simulink model "NavFilterTestHarness24"  (R2016b)
settings: Solver=FixedStepDiscrete  StartTime=startTime  StopTime=endTime  FixedStep=0.001  RelTol=1e-3  EnableMultiTasking=on
undefined symbols (not defined in the file): accel, ADSframe, ADStime, alignTime, angRate, ATTframe, CourseDeg, EAS2TAS, GndSpd, GPSframe, GPStime, Hgt, IMUframe, IMUtime, LatDeg, LngDeg, MagBiasX, MagBiasY, MagBiasZ, MAGframe, MAGtime, MagX, MagY, MagZ, msecHgtDelay, msecMagDelay, msecPosDelay, msecTasDelay, msecVelDelay, Pitch, Roll, Veas, VelD, Yaw
libraries: simulink x9, simulink_need_slupdate x2
(part 1 of 5)
settings Model: SimulationMode=rapid-accelerator  ExtModeTrigDuration=100  Creator=user  LastModifiedBy=lizarraga
settings DataIOCC: LimitDataPoints=on  SaveFinalState=on  SaveFormat=Array  SignalLoggingSaveFormat=ModelDataLogs  SaveOutput=off  SaveState=on  StateSaveName=tmp_raccel_xout
settings OptimizationCC: ExpressionDepthLimit=2147483647  EfficientMapNaN2IntZero=off  LifeSpan=inf
settings DebuggingCC: CheckSSInitialOutputMsg=off  UnderspecifiedInitializationDetection=Classic  MergeDetectMultiDrivingBlocksExec=none  SolverPrmCheckMsg=warning  ParameterPrecisionLossMsg=none  StateNameClashWarn=warning  SFUnexpectedBacktrackingDiag=warning  SFNoUnconditionalDefaultTransitionDiag=warning  SFExecutionAtInitializationDiag=none
settings HardwareCC: ProdBitPerPointer=32  ProdBitPerSizeT=32  ProdBitPerPtrDiffT=32  ProdLargestAtomicFloat=None  ProdIntDivRoundTo=Undefined  ProdEndianess=Unspecified  ProdWordSize=32  ProdHWDeviceType=32-bit Generic  TargetBitPerLong=64  TargetBitPerPointer=64  TargetBitPerSizeT=64  TargetBitPerPtrDiffT=64  TargetLongLongMode=on  TargetIntDivRoundTo=Zero  TargetEndianess=LittleEndian  TargetWordSize=64  TargetHWDeviceType=MATLAB Host  ProdEqTarget=off
settings ModelReferenceCC: PropagateSignalLabelsOutOfModel=off
settings SFSimCC: SimParseCustomCode=off
settings RTWCC: SystemTargetFile=raccel.tlc  TemplateMakefile=raccel_default_tmf  RTWVerbose=off  RTWUseSimCustomCode=on
settings CodeAppCC: GenerateComments=off  MaxIdLength=128  SimulinkBlockComments=off
settings RaccelTargetCC: ERTMultiwordTypeDef=System defined  ERTMultiwordLength=256  ParMdlRefBuildCompliant=off  GeneratePreprocessorConditionals=Disable all  ERTFirstTimeCompliant=off  MultiInstanceERTCode=off  ENABLE_SLEXEC_SSBRIDGE=0  RTWCAPISignals=off  RTWCAPIParams=off
settings ConfigComp: CovMetricSettings=dw  CovHtmlReporting=on  CovSaveCumulativeToWorkspaceVar=on  CovSaveSingleToWorkspaceVar=on  CovExternalEMLEnable=off

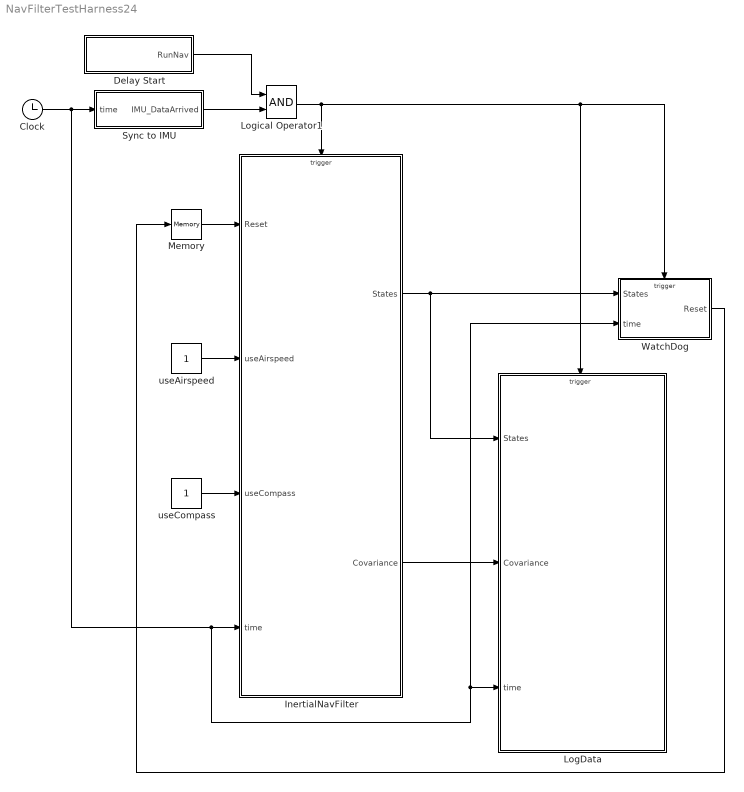
== system NavFilterTestHarness24 ==
  Clock : Clock
  Delay Start : Subsystem  TreatAsAtomicUnit=on  mask{navStartTime=alignTime}
      mask prompts: navStartTime "Nav Start Time"
  InertialNavFilter : Subsystem
  LogData : Subsystem
  Logical Operator1 : Logic  AllPortsSameDT=off  OutDataTypeStr=boolean
  Memory : Memory  InheritSampleTime=on
  Sync to IMU : Subsystem  TreatAsAtomicUnit=on
  WatchDog : Subsystem  TreatAsAtomicUnit=on
  useAirspeed : Constant  OutDataTypeStr=boolean
  useCompass : Constant  OutDataTypeStr=boolean
  wires:
  InertialNavFilter/1(States) -> LogData/1(States), WatchDog/1(States)
  Logical Operator1/1 -> LogData/Trigger, WatchDog/Trigger, InertialNavFilter/Trigger
  InertialNavFilter/2(Covariance) -> LogData/2(Covariance)
  WatchDog/1(Reset) -> Memory/1
  useAirspeed/1 -> InertialNavFilter/2(useAirspeed)
  useCompass/1 -> InertialNavFilter/3(useCompass)
  Clock/1 -> InertialNavFilter/4(time), LogData/3(time), WatchDog/2(time), Sync to IMU/1(time)
  Delay Start/1(RunNav) -> Logical Operator1/1
  Sync to IMU/1(IMU_DataArrived) -> Logical Operator1/2
  Memory/1 -> InertialNavFilter/1(Reset)

== system NavFilterTestHarness24/Delay Start ==
  Clock : Clock
  Compare To Constant2 : simulink/Logic and Bit Operations/Compare To Constant  relop=>  const=navStartTime  OutDataTypeStr=boolean
  RunNav : Outport
  wires:
  Clock/1 -> Compare To Constant2/1
  Compare To Constant2/1 -> RunNav/1

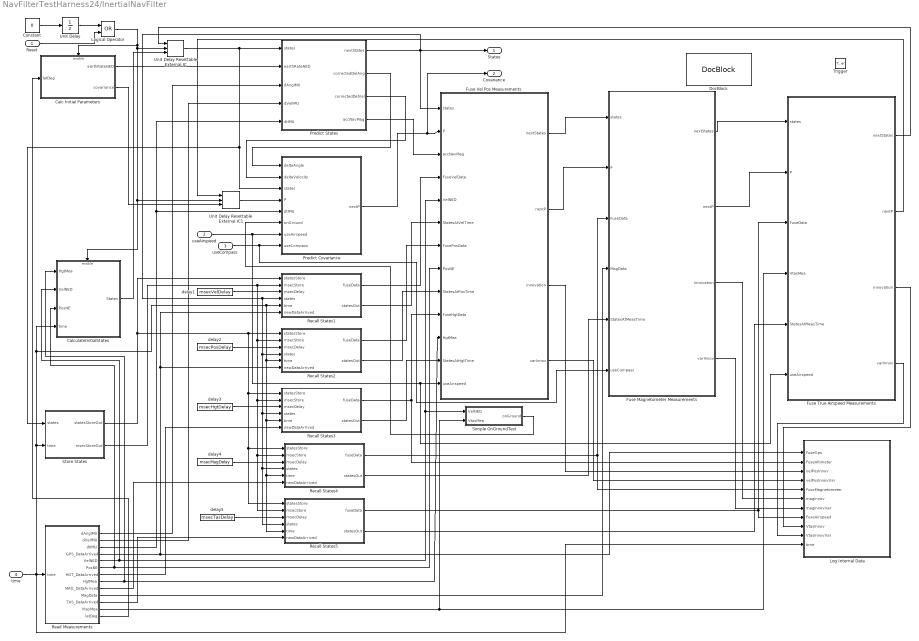
== system NavFilterTestHarness24/InertialNavFilter ==
  Reset : Inport  OutDataTypeStr=boolean  PortDimensions=1
  useAirspeed : Inport  Port=2  OutDataTypeStr=boolean  PortDimensions=1
  useCompass : Inport  Port=3  OutDataTypeStr=boolean  PortDimensions=1
  time : Inport  Port=4  OutDataTypeStr=double  PortDimensions=1
  Trigger : TriggerPort  VariantControl=Variant  PortDimensions=1
  Calc Initial Parameters : Subsystem
  CalculateInitialStates : Subsystem  TreatAsAtomicUnit=on
  Constant : Constant  Value=0  OutDataTypeStr=boolean
  DocBlock : simulink/Model-Wide Utilities/DocBlock  DocumentType=Text
      content=|
      | 24 State Extended Kalman Filter
      |
      | States :
      | 1 ... 4   : Quaternion parameters defining the rotation from local NED tangent frame to XYZ body axes
      | 5 ... 7   : North, East, Down velocity relative to and earth fixed reference point (m)
      | 8 ... 10  : North, East, Down position relative to and earth fixed reference point (m)
      | 11 ... 13 : IMU delta angle bias errors (rad)
      | 14 ... 16 : IMU delta velocity bias errors (m/s)
      | 17,18     : North, East wind velocity (m/s)
      | 19 ... 21 : North, East, Down earth magnetic field (same units as magnetometer output)
      | 22 ... 24 : X, Y, Z Body fixed magnetic field bias - opposite sign to APM offsets (same units as magnetometer output)
      |
      | Time Varying Parameters :
      | IMU delta angles (rad)
      | IMU delta velocity (rad)
      |
      | Observations :
      | North, East, Down velocity (m/s)
      | North, East position (m)
      | Height (m)
      | True Airspeed (m/s) - optional
      | X, Y, Z body fixed magnetic flux measurements (same units as magnetometer output) - optional
      |
      | Note : without compass/magnetometer measurements, the heading alignment cannot be maintained on the ground, so the filter will need to be re-started when flight commences.
  Fuse Magnetometer Measurements : MATLAB Function  TreatAsAtomicUnit=on
  Fuse True Airspeed Measurements : MATLAB Function  TreatAsAtomicUnit=on
  Fuse Vel Pos Measurements : MATLAB Function  TreatAsAtomicUnit=on
  Log Internal Data : Subsystem
  Logical Operator : Logic  Operator=OR  AllPortsSameDT=off  OutDataTypeStr=boolean
  Predict Covariance : MATLAB Function  TreatAsAtomicUnit=on
  Predict States : MATLAB Function  TreatAsAtomicUnit=on
  Read Measurements : Subsystem  TreatAsAtomicUnit=on
  Recall States1 : MATLAB Function  TreatAsAtomicUnit=on
  Recall States2 : MATLAB Function  TreatAsAtomicUnit=on
  Recall States3 : MATLAB Function  TreatAsAtomicUnit=on
  Recall States4 : MATLAB Function  TreatAsAtomicUnit=on
  Recall States5 : MATLAB Function  TreatAsAtomicUnit=on
  Simple OnGroundTest : Subsystem  TreatAsAtomicUnit=on
  Store States : MATLAB Function  TreatAsAtomicUnit=on
  Unit Delay : UnitDelay  InitialCondition=1  SampleTime=-1
  Unit Delay Resettable External IC : simulink_need_slupdate/Unit Delay Resettable External IC  tsamp=-1
  Unit Delay Resettable External IC1 : simulink_need_slupdate/Unit Delay Resettable External IC  tsamp=-1
  delay1 : Constant  Value=msecVelDelay  OutDataTypeStr=int32  SampleTime=-1
  delay2 : Constant  Value=msecPosDelay  OutDataTypeStr=int32  SampleTime=-1
  delay3 : Constant  Value=msecHgtDelay  OutDataTypeStr=int32  SampleTime=-1
  delay4 : Constant  Value=msecMagDelay  OutDataTypeStr=int32  SampleTime=-1
  delay5 : Constant  Value=msecTasDelay  OutDataTypeStr=int32  SampleTime=-1
  States : Outport  OutDataTypeStr=single  PortDimensions=24
  Covariance : Outport  Port=2  OutDataTypeStr=single  PortDimensions=[24,24]
  wires:
  CalculateInitialStates/1(States) -> Unit Delay Resettable External IC/3
  Unit Delay Resettable External IC/1 -> Predict States/1(states), Predict Covariance/3(states), Store States/1(states)
  Predict States/1(nextStates) -> States/1, Fuse Vel Pos Measurements/1(states), Recall States1/4(states), Recall States2/4(states), Recall States5/4(states), Recall States4/4(states), Recall States3/4(states)
  Unit Delay Resettable External IC1/1 -> Predict Covariance/4(P)
  Calc Initial Parameters/2(covariance) -> Unit Delay Resettable External IC1/3
  Predict States/2(correctedDelAng) -> Predict Covariance/1(deltaAngle)
  Predict States/3(correctedDelVel) -> Predict Covariance/2(deltaVelocity)
  Fuse Vel Pos Measurements/2(nextP) -> Fuse Magnetometer Measurements/2(P)
  Fuse Vel Pos Measurements/1(nextStates) -> Fuse Magnetometer Measurements/1(states)
  Fuse True Airspeed Measurements/2(nextP) -> Unit Delay Resettable External IC1/1
  Fuse True Airspeed Measurements/1(nextStates) -> Unit Delay Resettable External IC/1
  Fuse Magnetometer Measurements/1(nextStates) -> Fuse True Airspeed Measurements/1(states)
  Fuse Magnetometer Measurements/2(nextP) -> Fuse True Airspeed Measurements/2(P)
  Predict Covariance/1(nextP) -> Covariance/1, Fuse Vel Pos Measurements/2(P)
  Predict States/4(accNavMag) -> Fuse Vel Pos Measurements/3(accNavMag)
  Unit Delay/1 -> Logical Operator/1
  useCompass/1 -> Predict Covariance/8(useCompass), Fuse Magnetometer Measurements/6(useCompass)
  useAirspeed/1 -> Predict Covariance/7(useAirspeed), Fuse Vel Pos Measurements/13(useAirspeed), Fuse True Airspeed Measurements/6(useAirspeed)
  Fuse True Airspeed Measurements/3(innovation) -> Log Internal Data/9(VtasInnov)
  Fuse True Airspeed Measurements/4(varInnov) -> Log Internal Data/10(VtasInnovVar)
  Fuse Magnetometer Measurements/3(innovation) -> Log Internal Data/6(magInnov)
  Fuse Vel Pos Measurements/3(innovation) -> Log Internal Data/3(velPosInnov)
  Fuse Magnetometer Measurements/4(varInnov) -> Log Internal Data/7(magInnovVar)
  Fuse Vel Pos Measurements/4(varInnov) -> Log Internal Data/4(velPosInnovVar)
  time/1 -> Read Measurements/1(time), Log Internal Data/11(time), Store States/2(time), CalculateInitialStates/4(time), Recall States1/5(time), Recall States2/5(time), Recall States3/5(time), Recall States5/5(time), Recall States4/5(time)
  Simple OnGroundTest/1(onGround) -> Predict Covariance/6(onGround)
  Read Measurements/4(GPS_DataArrived) -> Log Internal Data/1(FuseGps), Recall States1/6(newDataArrived), Recall States2/6(newDataArrived)
  Read Measurements/5(VelNED) -> Simple OnGroundTest/1(VelNED), Fuse Vel Pos Measurements/5(VelNED), CalculateInitialStates/2(VelNED)
  Read Measurements/6(PosNE) -> CalculateInitialStates/3(PosNE), Fuse Vel Pos Measurements/8(PosNE)
  Read Measurements/8(HgtMea) -> CalculateInitialStates/1(HgtMea), Fuse Vel Pos Measurements/11(HgtMea)
  Read Measurements/10(MagData) -> Fuse Magnetometer Measurements/4(MagData)
  Read Measurements/12(VtasMea) -> Fuse True Airspeed Measurements/4(VtasMea), Simple OnGroundTest/2(VtasMea)
  Read Measurements/13(latDeg) -> Calc Initial Parameters/1(latDeg)
  Calc Initial Parameters/1(earthRateNED) -> Predict States/2(earthRateNED)
  Read Measurements/3(dtIMU) -> Predict Covariance/5(dtIMU), Predict States/5(dtIMU)
  Constant/1 -> Unit Delay/1
  Reset/1 -> Logical Operator/2
  Read Measurements/1(dAngIMU) -> Predict States/3(dAngIMU)
  Read Measurements/2(dVelIMU) -> Predict States/4(dVelIMU)
  Logical Operator/1 -> Unit Delay Resettable External IC/2, Unit Delay Resettable External IC1/2, CalculateInitialStates/Enable, Calc Initial Parameters/Enable
  Recall States1/2(statesOut) -> Fuse Vel Pos Measurements/6(StatesAtVelTime)
  Recall States1/1(fuseData) -> Fuse Vel Pos Measurements/4(FuseVelData)
  delay1/1 -> Recall States1/3(msecDelay)
  Store States/1(statesStoreOut) -> Recall States1/1(statesStore), Recall States2/1(statesStore), Recall States3/1(statesStore), Recall States4/1(statesStore), Recall States5/1(statesStore)
  Store States/2(msecStoreOut) -> Recall States1/2(msecStore), Recall States3/2(msecStore), Recall States4/2(msecStore), Recall States5/2(msecStore), Recall States2/2(msecStore)
  delay3/1 -> Recall States3/3(msecDelay)
  delay4/1 -> Recall States4/3(msecDelay)
  delay5/1 -> Recall States5/3(msecDelay)
  delay2/1 -> Recall States2/3(msecDelay)
  Read Measurements/7(HGT_DataArrived) -> Recall States3/6(newDataArrived)
  Read Measurements/9(MAG_DataArrived) -> Recall States4/6(newDataArrived)
  Read Measurements/11(TAS_DataArrived) -> Recall States5/6(newDataArrived)
  Recall States2/1(fuseData) -> Fuse Vel Pos Measurements/7(FusePosData)
  Recall States2/2(statesOut) -> Fuse Vel Pos Measurements/9(StatesAtPosTime)
  Recall States3/1(fuseData) -> Fuse Vel Pos Measurements/10(FuseHgtData), Log Internal Data/2(FuseAltimeter)
  Recall States3/2(statesOut) -> Fuse Vel Pos Measurements/12(StatesAtHgtTime)
  Recall States4/1(fuseData) -> Fuse Magnetometer Measurements/3(FuseData), Log Internal Data/5(FuseMagnetometer)
  Recall States4/2(statesOut) -> Fuse Magnetometer Measurements/5(StatesAtMeasTime)
  Recall States5/1(fuseData) -> Fuse True Airspeed Measurements/3(FuseData), Log Internal Data/8(FuseAirspeed)
  Recall States5/2(statesOut) -> Fuse True Airspeed Measurements/5(StatesAtMeasTime)

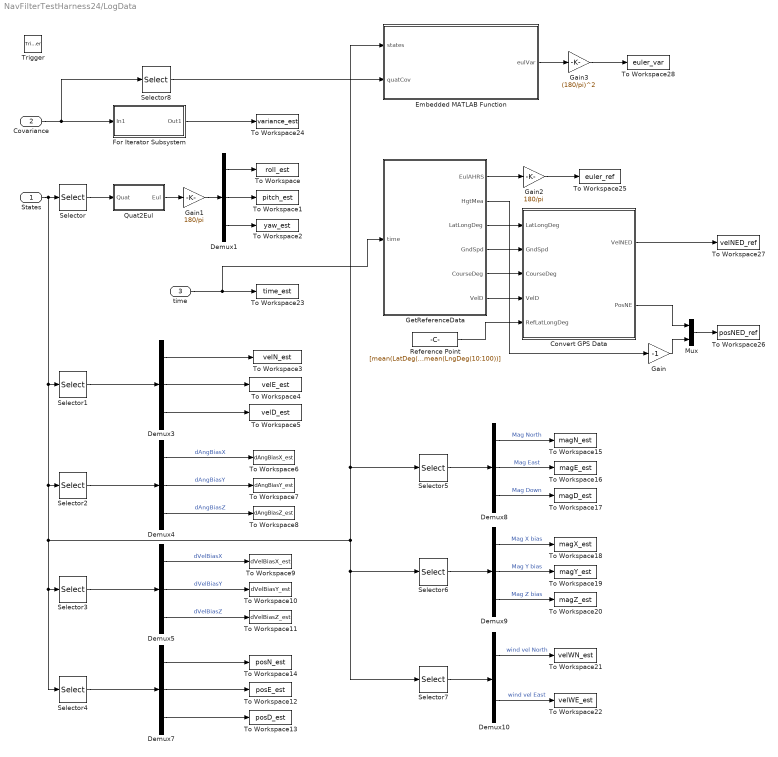
== system NavFilterTestHarness24/LogData ==
  States : Inport
  Covariance : Inport  Port=2  PortDimensions=[24,24]
  time : Inport  Port=3  OutDataTypeStr=double  PortDimensions=1
  Trigger : TriggerPort  VariantControl=Variant  PortDimensions=1
  Convert GPS Data : MATLAB Function  TreatAsAtomicUnit=on
  Demux{1,3..5,7..9} (7 alike) : Demux  Outputs=3
  Demux10 : Demux  Outputs=2
  Embedded MATLAB Function : MATLAB Function  TreatAsAtomicUnit=on
  For Iterator Subsystem : Subsystem  TreatAsAtomicUnit=on
  Gain : Gain  Gain=-1
  Gain1 : Gain  Gain=180/pi
  Gain2 : Gain  Gain=180/pi
  Gain3 : Gain  Gain=(180/pi)^2
  GetReferenceData : Subsystem  TreatAsAtomicUnit=on
  Mux : Mux  Inputs=2
  Quat2Eul : Subsystem
  Reference Point : Constant  Value=[mean(LatDeg(10:100)),mean(LngDeg(10:100))]  OutDataTypeStr=single
  Selector : Selector  InputPortWidth=24  IndexOptions=Index vector (dialog)  Indices=[1:4]  OutputSizes=1
  Selector1 : Selector  InputPortWidth=24  IndexOptions=Index vector (dialog)  Indices=[5:7]  OutputSizes=1
  Selector2 : Selector  InputPortWidth=24  IndexOptions=Index vector (dialog)  Indices=[11:13]  OutputSizes=1
  Selector3 : Selector  InputPortWidth=24  IndexOptions=Index vector (dialog)  Indices=[14:16]  OutputSizes=1
  Selector4 : Selector  InputPortWidth=24  IndexOptions=Index vector (dialog)  Indices=[8:10]  OutputSizes=1
  Selector5 : Selector  InputPortWidth=24  IndexOptions=Index vector (dialog)  Indices=[19:21]  OutputSizes=1
  Selector6 : Selector  InputPortWidth=24  IndexOptions=Index vector (dialog)  Indices=[22:24]  OutputSizes=1
  Selector7 : Selector  InputPortWidth=24  IndexOptions=Index vector (dialog)  Indices=[17:18]  OutputSizes=1
  Selector8 : Selector  NumberOfDimensions=2  InputPortWidth=3  IndexOptions=Index vector (dialog),Index vector (dialog)  Indices=[1:4],[1:4]  OutputSizes=1,1
  To Workspace : ToWorkspace  VariableName=roll_est  SampleTime=-1
  To Workspace1 : ToWorkspace  VariableName=pitch_est  SampleTime=-1
  To Workspace10 : ToWorkspace  VariableName=dVelBiasY_est  SampleTime=-1
  To Workspace11 : ToWorkspace  VariableName=dVelBiasZ_est  SampleTime=-1
  To Workspace12 : ToWorkspace  VariableName=posE_est  SampleTime=-1
  To Workspace13 : ToWorkspace  VariableName=posD_est  SampleTime=-1
  To Workspace14 : ToWorkspace  VariableName=posN_est  SampleTime=-1
  To Workspace15 : ToWorkspace  VariableName=magN_est  SampleTime=-1
  To Workspace16 : ToWorkspace  VariableName=magE_est  SampleTime=-1
  To Workspace17 : ToWorkspace  VariableName=magD_est  SampleTime=-1
  To Workspace18 : ToWorkspace  VariableName=magX_est  SampleTime=-1
  To Workspace19 : ToWorkspace  VariableName=magY_est  SampleTime=-1
  To Workspace2 : ToWorkspace  VariableName=yaw_est  SampleTime=-1
  To Workspace20 : ToWorkspace  VariableName=magZ_est  SampleTime=-1
  To Workspace21 : ToWorkspace  VariableName=velWN_est  SampleTime=-1
  To Workspace22 : ToWorkspace  VariableName=velWE_est  SampleTime=-1
  To Workspace23 : ToWorkspace  VariableName=time_est  SampleTime=-1
  To Workspace24 : ToWorkspace  VariableName=variance_est  SampleTime=-1
  To Workspace25 : ToWorkspace  VariableName=euler_ref  SampleTime=-1
  To Workspace26 : ToWorkspace  VariableName=posNED_ref  SampleTime=-1
  To Workspace27 : ToWorkspace  VariableName=velNED_ref  SampleTime=-1
  To Workspace28 : ToWorkspace  VariableName=euler_var  SampleTime=-1
  To Workspace3 : ToWorkspace  VariableName=velN_est  SampleTime=-1
  To Workspace4 : ToWorkspace  VariableName=velE_est  SampleTime=-1
  To Workspace5 : ToWorkspace  VariableName=velD_est  SampleTime=-1
  To Workspace6 : ToWorkspace  VariableName=dAngBiasX_est  SampleTime=-1
  To Workspace7 : ToWorkspace  VariableName=dAngBiasY_est  SampleTime=-1
  To Workspace8 : ToWorkspace  VariableName=dAngBiasZ_est  SampleTime=-1
  To Workspace9 : ToWorkspace  VariableName=dVelBiasX_est  SampleTime=-1
  wires:
  Quat2Eul/1(Eul) -> Gain1/1
  Selector/1 -> Quat2Eul/1(Quat)
  States/1 -> Selector2/1, Selector4/1, Selector3/1, Embedded MATLAB Function/1(states), Selector5/1, Selector6/1, Selector7/1, Selector1/1, Selector/1
  Gain1/1 -> Demux1/1
  Selector2/1 -> Demux4/1
  Selector3/1 -> Demux5/1
  Demux4/1 -> To Workspace6/1  "dAngBiasX"
  Selector4/1 -> Demux7/1
  Selector5/1 -> Demux8/1
  Selector6/1 -> Demux9/1
  Selector7/1 -> Demux10/1
  Demux4/3 -> To Workspace8/1  "dAngBiasZ"
  Demux4/2 -> To Workspace7/1  "dAngBiasY"
  Demux5/1 -> To Workspace9/1  "dVelBiasX"
  Demux5/2 -> To Workspace10/1  "dVelBiasY"
  Demux5/3 -> To Workspace11/1  "dVelBiasZ"
  Demux8/1 -> To Workspace15/1  "Mag North"
  Demux8/2 -> To Workspace16/1  "Mag East"
  Demux8/3 -> To Workspace17/1  "Mag Down"
  Demux9/1 -> To Workspace18/1  "Mag X bias"
  Demux9/2 -> To Workspace19/1  "Mag Y bias"
  Demux9/3 -> To Workspace20/1  "Mag Z bias"
  Demux10/1 -> To Workspace21/1  "wind vel North"
  Demux10/2 -> To Workspace22/1  "wind vel East"
  time/1 -> To Workspace23/1, GetReferenceData/1(time)
  Demux7/1 -> To Workspace14/1
  Demux7/2 -> To Workspace12/1
  Demux7/3 -> To Workspace13/1
  Demux3/1 -> To Workspace3/1
  Demux3/2 -> To Workspace4/1
  Demux3/3 -> To Workspace5/1
  Demux1/3 -> To Workspace2/1
  Demux1/2 -> To Workspace1/1
  Demux1/1 -> To Workspace/1
  Covariance/1 -> Selector8/1, For Iterator Subsystem/1(In1)
  GetReferenceData/1(EulAHRS) -> Gain2/1
  GetReferenceData/2(HgtMea) -> Gain/1
  Convert GPS Data/2(PosNE) -> Mux/1
  Mux/1 -> To Workspace26/1
  Gain/1 -> Mux/2
  Gain2/1 -> To Workspace25/1
  Embedded MATLAB Function/1(eulVar) -> Gain3/1
  For Iterator Subsystem/1(Out1) -> To Workspace24/1
  Selector8/1 -> Embedded MATLAB Function/2(quatCov)
  Gain3/1 -> To Workspace28/1
  Selector1/1 -> Demux3/1
  GetReferenceData/3(LatLongDeg) -> Convert GPS Data/1(LatLongDeg)
  GetReferenceData/4(GndSpd) -> Convert GPS Data/2(GndSpd)
  GetReferenceData/5(CourseDeg) -> Convert GPS Data/3(CourseDeg)
  GetReferenceData/6(VelD) -> Convert GPS Data/4(VelD)
  Reference Point/1 -> Convert GPS Data/5(RefLatLongDeg)
  Convert GPS Data/1(VelNED) -> To Workspace27/1

== system NavFilterTestHarness24/Sync to IMU ==
  time : Inport
  Detect Change1 : simulink/Logic and Bit Operations/Detect Change  vinit=0  InputProcessing=Inherited  OutDataTypeStr=boolean
  Lookup Frame Counter : Lookup_n-D  NumberOfTableDimensions=1  BreakpointsForDimension1=IMUtime  BeginIndexSearchUsingPreviousIndexResult=on  Table=IMUframe  InterpMethod=Flat  DiagnosticForOutOfRangeInput=Error  RndMeth=Simplest  InputSameDT=on
  IMU_DataArrived : Outport  OutDataTypeStr=boolean
  wires:
  Lookup Frame Counter/1 -> Detect Change1/1
  time/1 -> Lookup Frame Counter/1
  Detect Change1/1 -> IMU_DataArrived/1

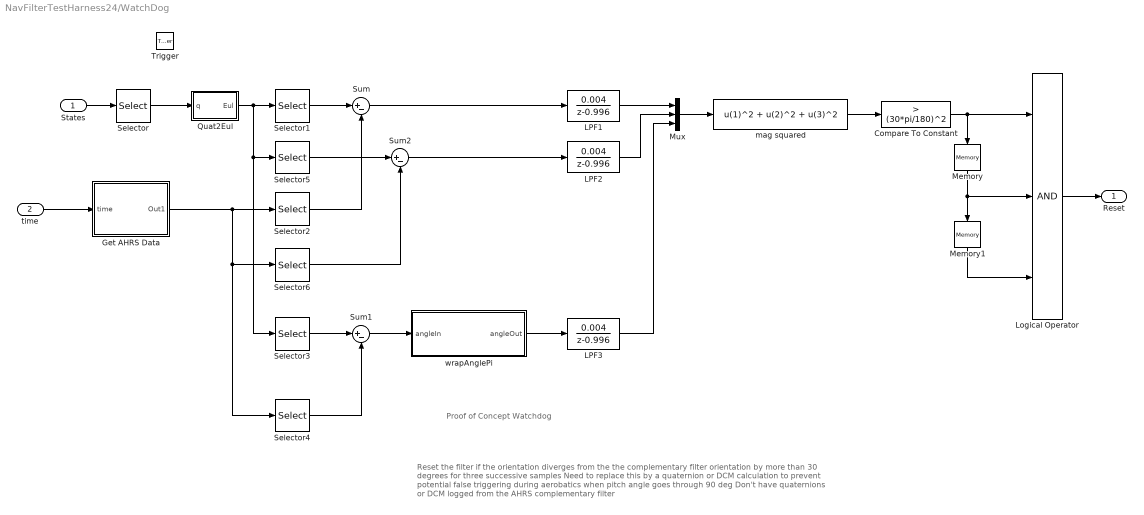
== system NavFilterTestHarness24/WatchDog ==
  note: Reset the filter if the orientation diverges from the the complementary filter orientation  by more than 30 degrees for three successive samples
      | Need to replace this by a quaternion or DCM calculation to prevent potential false triggering during aerobatics when pitch angle goes through 90 deg
      | Don't have quaternions or DCM logged from the AHRS complementary filter
  note: Proof of Concept Watchdog
  States : Inport
  time : Inport  Port=2
  Trigger : TriggerPort  VariantControl=Variant  PortDimensions=1
  Compare To Constant : simulink/Logic and Bit Operations/Compare To Constant  relop=>  const=(30*pi/180)^2  OutDataTypeStr=boolean
  Get AHRS Data : Subsystem
  LPF1 : DiscreteTransferFcn  Numerator=0.004  Denominator=[1 -0.996]
  LPF2 : DiscreteTransferFcn  Numerator=0.004  Denominator=[1 -0.996]
  LPF3 : DiscreteTransferFcn  Numerator=0.004  Denominator=[1 -0.996]
  Logical Operator : Logic  Inputs=3  AllPortsSameDT=off  OutDataTypeStr=boolean
  Memory : Memory  InheritSampleTime=on
  Memory1 : Memory  InheritSampleTime=on
  Mux : Mux  Inputs=3
  Quat2Eul : Subsystem
  Selector : Selector  InputPortWidth=24  IndexOptions=Index vector (dialog)  Indices=[1:4]  OutputSizes=1
  Selector1 : Selector  InputPortWidth=3  IndexOptions=Index vector (dialog)  Indices=1  OutputSizes=1
  Selector2 : Selector  InputPortWidth=3  IndexOptions=Index vector (dialog)  Indices=1  OutputSizes=1
  Selector3 : Selector  InputPortWidth=3  IndexOptions=Index vector (dialog)  Indices=3  OutputSizes=1
  Selector4 : Selector  InputPortWidth=3  IndexOptions=Index vector (dialog)  Indices=3  OutputSizes=1
  Selector5 : Selector  InputPortWidth=3  IndexOptions=Index vector (dialog)  Indices=2  OutputSizes=1
  Selector6 : Selector  InputPortWidth=3  IndexOptions=Index vector (dialog)  Indices=2  OutputSizes=1
  Sum : Sum  Inputs=|+-
  Sum1 : Sum  Inputs=|+-
  Sum2 : Sum  Inputs=|+-
  mag squared : Fcn  Expr=u(1)^2 + u(2)^2 + u(3)^2
  wrapAnglePi : MATLAB Function  TreatAsAtomicUnit=on
  Reset : Outport  OutDataTypeStr=boolean  PortDimensions=1
  wires:
  Selector/1 -> Quat2Eul/1(q)
  States/1 -> Selector/1
  Quat2Eul/1(Eul) -> Selector1/1, Selector3/1, Selector5/1
  Get AHRS Data/1(Out1) -> Selector2/1, Selector4/1, Selector6/1
  Selector3/1 -> Sum1/1
  Selector4/1 -> Sum1/2
  Sum1/1 -> wrapAnglePi/1(angleIn)
  Sum/1 -> LPF1/1
  wrapAnglePi/1(angleOut) -> LPF3/1
  Mux/1 -> mag squared/1
  mag squared/1 -> Compare To Constant/1
  Compare To Constant/1 -> Logical Operator/1, Memory/1
  Logical Operator/1 -> Reset/1
  Memory/1 -> Logical Operator/2, Memory1/1
  Memory1/1 -> Logical Operator/3
  Selector1/1 -> Sum/1
  Selector2/1 -> Sum/2
  Selector5/1 -> Sum2/1
  Selector6/1 -> Sum2/2
  Sum2/1 -> LPF2/1
  LPF1/1 -> Mux/1
  LPF2/1 -> Mux/2
  LPF3/1 -> Mux/3
  time/1 -> Get AHRS Data/1(time)

== system NavFilterTestHarness24/InertialNavFilter/Calc Initial Parameters ==
  latDeg : Inport  OutDataTypeStr=single  PortDimensions=1
  Enable : EnablePort
  Embedded MATLAB Function : MATLAB Function  TreatAsAtomicUnit=on
  earthRateNED : Outport  PortDimensions=3
  covariance : Outport  Port=2
  wires:
  Embedded MATLAB Function/2(covariance) -> covariance/1
  Embedded MATLAB Function/1(earthRateNED) -> earthRateNED/1
  latDeg/1 -> Embedded MATLAB Function/1(latDeg)

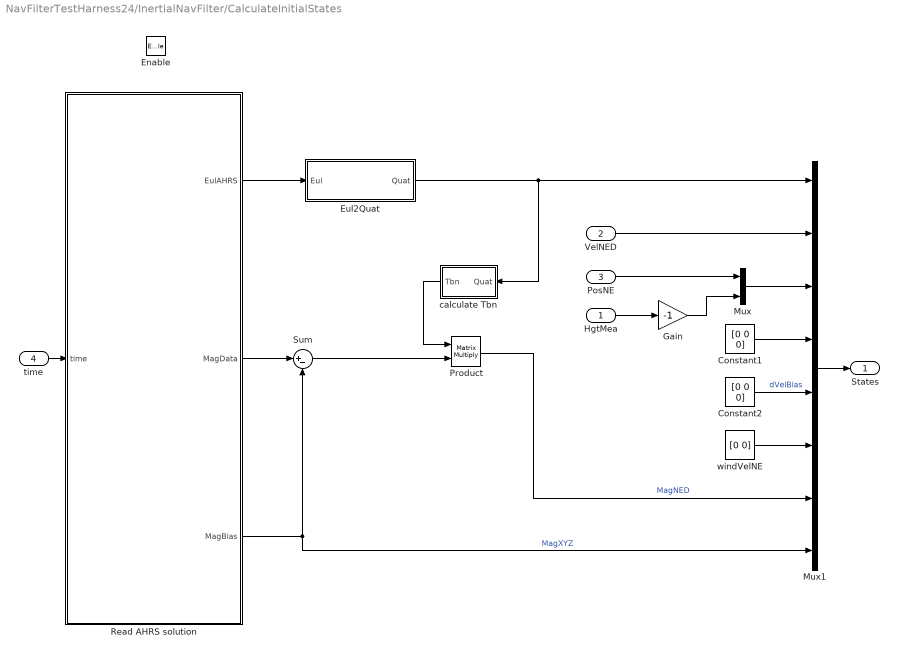
== system NavFilterTestHarness24/InertialNavFilter/CalculateInitialStates ==
  HgtMea : Inport
  VelNED : Inport  Port=2  OutDataTypeStr=single
  PosNE : Inport  Port=3
  time : Inport  Port=4
  Enable : EnablePort
  Constant1 : Constant  Value=[0 0 0]  OutDataTypeStr=single
  Constant2 : Constant  Value=[0 0 0]  OutDataTypeStr=single
  Eul2Quat : Subsystem
  Gain : Gain  Gain=-1
  Mux : Mux  Inputs=2
  Mux1 : Mux  Inputs=8
  Product : Product  Multiplication=Matrix(*)  RndMeth=Zero
  Read AHRS solution : Subsystem  TreatAsAtomicUnit=on
  Sum : Sum  Inputs=|+-
  calculate Tbn : Subsystem
  windVelNE : Constant  Value=[0 0]  OutDataTypeStr=single
  States : Outport
  wires:
  Sum/1 -> Product/2
  Eul2Quat/1(Quat) -> calculate Tbn/1(Quat), Mux1/1
  Mux1/1 -> States/1
  windVelNE/1 -> Mux1/6
  Constant2/1 -> Mux1/5  "dVelBias"
  VelNED/1 -> Mux1/2
  Product/1 -> Mux1/7  "MagNED"
  Gain/1 -> Mux/2
  PosNE/1 -> Mux/1
  Mux/1 -> Mux1/3
  Constant1/1 -> Mux1/4
  HgtMea/1 -> Gain/1
  Read AHRS solution/1(EulAHRS) -> Eul2Quat/1(Eul)
  Read AHRS solution/2(MagData) -> Sum/1
  Read AHRS solution/3(MagBias) -> Sum/2, Mux1/8  "MagXYZ"
  calculate Tbn/1(Tbn) -> Product/1
  time/1 -> Read AHRS solution/1(time)

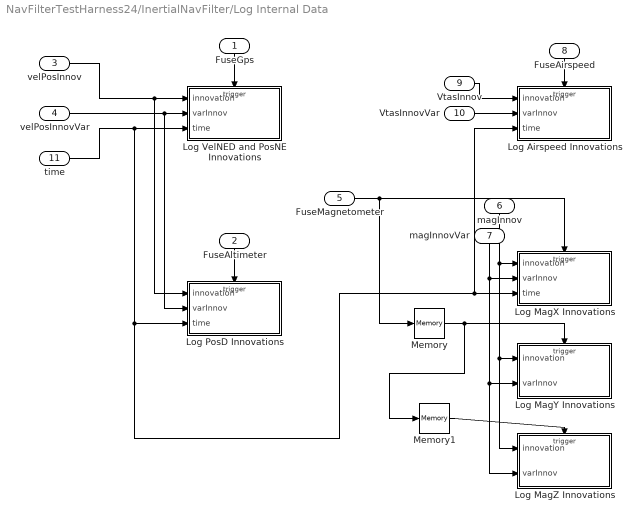
== system NavFilterTestHarness24/InertialNavFilter/Log Internal Data ==
  FuseGps : Inport
  FuseAltimeter : Inport  Port=2
  velPosInnov : Inport  Port=3
  velPosInnovVar : Inport  Port=4
  FuseMagnetometer : Inport  Port=5
  magInnov : Inport  Port=6
  magInnovVar : Inport  Port=7
  FuseAirspeed : Inport  Port=8
  VtasInnov : Inport  Port=9
  VtasInnovVar : Inport  Port=10
  time : Inport  Port=11
  Log Airspeed Innovations : Subsystem
  Log MagX Innovations : Subsystem
  Log MagY Innovations : Subsystem
  Log MagZ Innovations : Subsystem
  Log PosD Innovations : Subsystem
  Log VelNED and PosNE Innovations : Subsystem
  Memory : Memory  InheritSampleTime=on
  Memory1 : Memory  InheritSampleTime=on
  wires:
  magInnov/1 -> Log MagZ Innovations/1(innovation), Log MagY Innovations/1(innovation), Log MagX Innovations/1(innovation)
  magInnovVar/1 -> Log MagY Innovations/2(varInnov), Log MagZ Innovations/2(varInnov), Log MagX Innovations/2(varInnov)
  time/1 -> Log VelNED and PosNE Innovations/3(time), Log PosD Innovations/3(time), Log MagX Innovations/3(time), Log Airspeed Innovations/3(time)
  Memory1/1 -> Log MagZ Innovations/Trigger
  Memory/1 -> Log MagY Innovations/Trigger, Memory1/1
  FuseMagnetometer/1 -> Memory/1, Log MagX Innovations/Trigger
  velPosInnov/1 -> Log PosD Innovations/1(innovation), Log VelNED and PosNE Innovations/1(innovation)
  velPosInnovVar/1 -> Log PosD Innovations/2(varInnov), Log VelNED and PosNE Innovations/2(varInnov)
  FuseGps/1 -> Log VelNED and PosNE Innovations/Trigger
  FuseAltimeter/1 -> Log PosD Innovations/Trigger
  FuseAirspeed/1 -> Log Airspeed Innovations/Trigger
  VtasInnov/1 -> Log Airspeed Innovations/1(innovation)
  VtasInnovVar/1 -> Log Airspeed Innovations/2(varInnov)

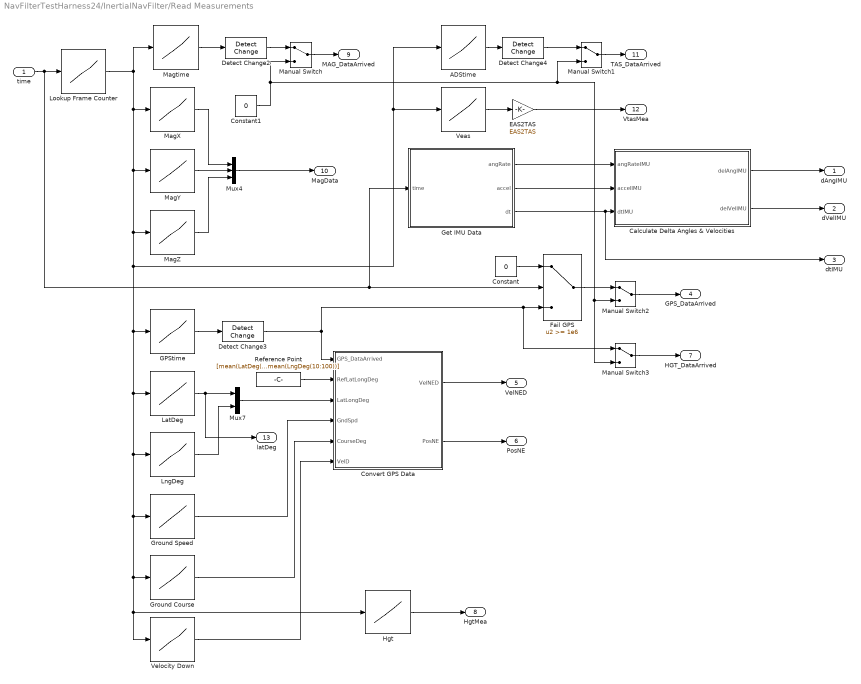
== system NavFilterTestHarness24/InertialNavFilter/Read Measurements ==
  time : Inport
  ADStime : Lookup_n-D  NumberOfTableDimensions=1  BreakpointsForDimension1=ADSframe  BeginIndexSearchUsingPreviousIndexResult=on  Table=ADStime  InterpMethod=Flat  OutDataTypeStr=single  RndMeth=Simplest  InputSameDT=on
  Calculate Delta Angles & Velocities : MATLAB Function  TreatAsAtomicUnit=on
  Constant : Constant  Value=0  OutDataTypeStr=boolean
  Constant1 : Constant  Value=0  OutDataTypeStr=boolean
  Convert GPS Data : MATLAB Function  TreatAsAtomicUnit=on
  Detect Change2 : simulink/Logic and Bit Operations/Detect Change  vinit=0  InputProcessing=Inherited  OutDataTypeStr=boolean
  Detect Change3 : simulink/Logic and Bit Operations/Detect Change  vinit=0  InputProcessing=Inherited  OutDataTypeStr=boolean
  Detect Change4 : simulink/Logic and Bit Operations/Detect Change  vinit=0  InputProcessing=Inherited  OutDataTypeStr=boolean
  EAS2TAS : Gain  Gain=EAS2TAS
  Fail GPS : Switch  Threshold=1e6
  GPStime : Lookup_n-D  NumberOfTableDimensions=1  BreakpointsForDimension1=GPSframe  BeginIndexSearchUsingPreviousIndexResult=on  Table=GPStime  InterpMethod=Flat  OutDataTypeStr=single  RndMeth=Simplest  InputSameDT=on
  Get IMU Data : Subsystem  TreatAsAtomicUnit=on
  Ground Course : Lookup_n-D  NumberOfTableDimensions=1  BreakpointsForDimension1=GPSframe  BeginIndexSearchUsingPreviousIndexResult=on  Table=CourseDeg  InterpMethod=Flat  OutDataTypeStr=single  RndMeth=Simplest  InputSameDT=on
  Ground Speed : Lookup_n-D  NumberOfTableDimensions=1  BreakpointsForDimension1=GPSframe  BeginIndexSearchUsingPreviousIndexResult=on  Table=GndSpd  InterpMethod=Flat  OutDataTypeStr=single  RndMeth=Simplest  InputSameDT=on
  Hgt : Lookup_n-D  NumberOfTableDimensions=1  BreakpointsForDimension1=GPSframe  BeginIndexSearchUsingPreviousIndexResult=on  Table=Hgt  InterpMethod=Flat  OutDataTypeStr=single  RndMeth=Simplest  InputSameDT=on
  LatDeg : Lookup_n-D  NumberOfTableDimensions=1  BreakpointsForDimension1=GPSframe  BeginIndexSearchUsingPreviousIndexResult=on  Table=LatDeg  InterpMethod=Flat  OutDataTypeStr=single  RndMeth=Simplest  InputSameDT=on
  LngDeg : Lookup_n-D  NumberOfTableDimensions=1  BreakpointsForDimension1=GPSframe  BeginIndexSearchUsingPreviousIndexResult=on  Table=LngDeg  InterpMethod=Flat  OutDataTypeStr=single  RndMeth=Simplest  InputSameDT=on
  Lookup Frame Counter : Lookup_n-D  NumberOfTableDimensions=1  BreakpointsForDimension1=IMUtime  BeginIndexSearchUsingPreviousIndexResult=on  Table=IMUframe  InterpMethod=Flat  DiagnosticForOutOfRangeInput=Error  RndMeth=Simplest  InputSameDT=on
  MagX : Lookup_n-D  NumberOfTableDimensions=1  BreakpointsForDimension1=MAGframe  BeginIndexSearchUsingPreviousIndexResult=on  Table=MagX  InterpMethod=Flat  OutDataTypeStr=single  RndMeth=Simplest  InputSameDT=on
  MagY : Lookup_n-D  NumberOfTableDimensions=1  BreakpointsForDimension1=MAGframe  BeginIndexSearchUsingPreviousIndexResult=on  Table=MagY  InterpMethod=Flat  OutDataTypeStr=single  RndMeth=Simplest  InputSameDT=on
  MagZ : Lookup_n-D  NumberOfTableDimensions=1  BreakpointsForDimension1=MAGframe  BeginIndexSearchUsingPreviousIndexResult=on  Table=MagZ  InterpMethod=Flat  OutDataTypeStr=single  RndMeth=Simplest  InputSameDT=on
  Magtime : Lookup_n-D  NumberOfTableDimensions=1  BreakpointsForDimension1=MAGframe  BeginIndexSearchUsingPreviousIndexResult=on  Table=MAGtime  InterpMethod=Flat  OutDataTypeStr=single  RndMeth=Simplest  InputSameDT=on
  Manual Switch{,1..3} (4 alike) : ManualSwitch
  Mux4 : Mux  Inputs=3
  Mux7 : Mux  Inputs=2
  Reference Point : Constant  Value=[mean(LatDeg(10:100)),mean(LngDeg(10:100))]  OutDataTypeStr=single
  Veas : Lookup_n-D  NumberOfTableDimensions=1  BreakpointsForDimension1=ADSframe  BeginIndexSearchUsingPreviousIndexResult=on  Table=Veas  InterpMethod=Flat  OutDataTypeStr=single  RndMeth=Simplest  InputSameDT=on
  Velocity Down : Lookup_n-D  NumberOfTableDimensions=1  BreakpointsForDimension1=GPSframe  BeginIndexSearchUsingPreviousIndexResult=on  Table=VelD  InterpMethod=Flat  OutDataTypeStr=single  RndMeth=Simplest  InputSameDT=on
  dAngIMU : Outport
  dVelIMU : Outport  Port=2
  dtIMU : Outport  Port=3
  GPS_DataArrived : Outport  Port=4  OutDataTypeStr=boolean
  VelNED : Outport  Port=5  OutDataTypeStr=single
  PosNE : Outport  Port=6  OutDataTypeStr=single
  HGT_DataArrived : Outport  Port=7  OutDataTypeStr=boolean
  HgtMea : Outport  Port=8  OutDataTypeStr=single
  MAG_DataArrived : Outport  Port=9  OutDataTypeStr=boolean
  MagData : Outport  Port=10  OutDataTypeStr=single
  TAS_DataArrived : Outport  Port=11  OutDataTypeStr=boolean
  VtasMea : Outport  Port=12  OutDataTypeStr=single
  latDeg : Outport  Port=13  OutDataTypeStr=single
  wires:
  Lookup Frame Counter/1 -> MagX/1, MagY/1, MagZ/1, LatDeg/1, LngDeg/1, Ground Course/1, Velocity Down/1, Hgt/1, Ground Speed/1, GPStime/1, ADStime/1, Veas/1, Magtime/1
  Mux4/1 -> MagData/1
  MagY/1 -> Mux4/2
  MagX/1 -> Mux4/1
  MagZ/1 -> Mux4/3
  Veas/1 -> EAS2TAS/1
  Manual Switch/1 -> MAG_DataArrived/1
  EAS2TAS/1 -> VtasMea/1
  Manual Switch1/1 -> TAS_DataArrived/1
  time/1 -> Lookup Frame Counter/1, Fail GPS/2, Get IMU Data/1(time)
  LatDeg/1 -> Mux7/1, latDeg/1
  LngDeg/1 -> Mux7/2
  Hgt/1 -> HgtMea/1
  Magtime/1 -> Detect Change2/1
  Mux7/1 -> Convert GPS Data/3(LatLongDeg)
  GPStime/1 -> Detect Change3/1
  Detect Change3/1 -> Convert GPS Data/1(GPS_DataArrived), Fail GPS/3, Manual Switch3/1
  Ground Speed/1 -> Convert GPS Data/4(GndSpd)
  Ground Course/1 -> Convert GPS Data/5(CourseDeg)
  Velocity Down/1 -> Convert GPS Data/6(VelD)
  Reference Point/1 -> Convert GPS Data/2(RefLatLongDeg)
  Detect Change2/1 -> Manual Switch/1
  Constant1/1 -> Manual Switch/2, Manual Switch1/2, Manual Switch2/2, Manual Switch3/2
  Convert GPS Data/1(VelNED) -> VelNED/1
  Convert GPS Data/2(PosNE) -> PosNE/1
  ADStime/1 -> Detect Change4/1
  Detect Change4/1 -> Manual Switch1/1
  Constant/1 -> Fail GPS/1
  Fail GPS/1 -> Manual Switch2/1
  Manual Switch2/1 -> GPS_DataArrived/1
  Manual Switch3/1 -> HGT_DataArrived/1
  Get IMU Data/2(accel) -> Calculate Delta Angles & Velocities/2(accelIMU)
  Get IMU Data/3(dt) -> Calculate Delta Angles & Velocities/3(dtIMU), dtIMU/1
  Calculate Delta Angles & Velocities/1(delAngIMU) -> dAngIMU/1
  Calculate Delta Angles & Velocities/2(delVelIMU) -> dVelIMU/1
  Get IMU Data/1(angRate) -> Calculate Delta Angles & Velocities/1(angRateIMU)

== system NavFilterTestHarness24/InertialNavFilter/Simple OnGroundTest ==
  VelNED : Inport
  VtasMea : Inport  Port=2
  Logical Operator : Logic  AllPortsSameDT=off  OutDataTypeStr=boolean
  Test Airspeed : simulink/Logic and Bit Operations/Compare To Constant  relop=<  const=8  OutDataTypeStr=boolean
  Test Ground Spee : simulink/Logic and Bit Operations/Compare To Constant  relop=<  const=2  OutDataTypeStr=boolean
  gndSpd : Fcn  Expr=sqrt(u(1)^2 + u(2)^2)
  onGround : Outport
  wires:
  gndSpd/1 -> Test Ground Spee/1
  Test Airspeed/1 -> Logical Operator/2
  Test Ground Spee/1 -> Logical Operator/1
  VelNED/1 -> gndSpd/1
  VtasMea/1 -> Test Airspeed/1
  Logical Operator/1 -> onGround/1

== system NavFilterTestHarness24/LogData/For Iterator Subsystem ==
  In1 : Inport
  Assignment : Assignment  OutputInitialize=Specify size for each dimension in table  IndexOptions=Index vector (port)  Indices=1  OutputSizes=24
  For Iterator : ForIterator  IterationLimit=24
  Select5 : Selector  NumberOfDimensions=2  InputPortWidth=3  IndexOptions=Index vector (port),Index vector (port)  Indices=1,1  OutputSizes=1,1
  Out1 : Outport
  wires:
  In1/1 -> Select5/1
  For Iterator/1 -> Select5/2, Select5/3, Assignment/2
  Select5/1 -> Assignment/1
  Assignment/1 -> Out1/1

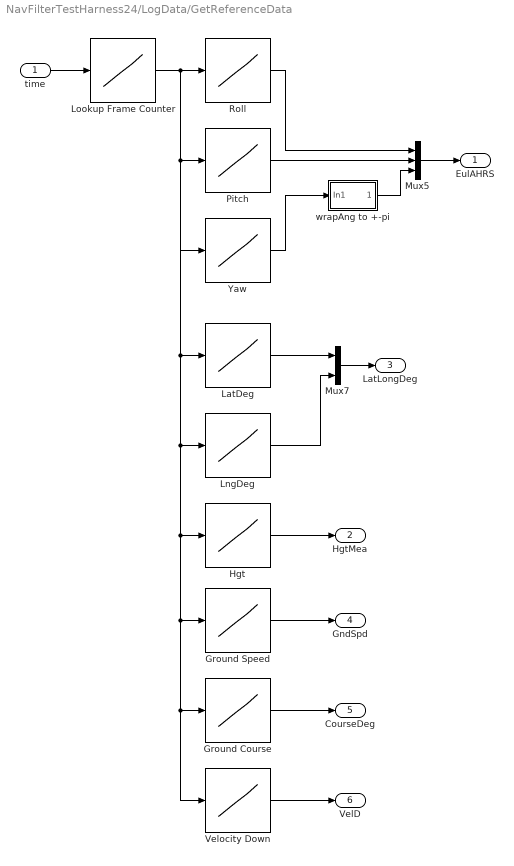
== system NavFilterTestHarness24/LogData/GetReferenceData ==
  time : Inport
  Ground Course : Lookup_n-D  NumberOfTableDimensions=1  BreakpointsForDimension1=GPSframe  BeginIndexSearchUsingPreviousIndexResult=on  Table=CourseDeg  InterpMethod=Flat  OutDataTypeStr=single  RndMeth=Simplest  InputSameDT=on
  Ground Speed : Lookup_n-D  NumberOfTableDimensions=1  BreakpointsForDimension1=GPSframe  BeginIndexSearchUsingPreviousIndexResult=on  Table=GndSpd  InterpMethod=Flat  OutDataTypeStr=single  RndMeth=Simplest  InputSameDT=on
  Hgt : Lookup_n-D  NumberOfTableDimensions=1  BreakpointsForDimension1=GPSframe  BeginIndexSearchUsingPreviousIndexResult=on  Table=Hgt  InterpMethod=Flat  OutDataTypeStr=single  RndMeth=Simplest  InputSameDT=on
  LatDeg : Lookup_n-D  NumberOfTableDimensions=1  BreakpointsForDimension1=GPSframe  BeginIndexSearchUsingPreviousIndexResult=on  Table=LatDeg  InterpMethod=Flat  OutDataTypeStr=single  RndMeth=Simplest  InputSameDT=on
  LngDeg : Lookup_n-D  NumberOfTableDimensions=1  BreakpointsForDimension1=GPSframe  BeginIndexSearchUsingPreviousIndexResult=on  Table=LngDeg  InterpMethod=Flat  OutDataTypeStr=single  RndMeth=Simplest  InputSameDT=on
  Lookup Frame Counter : Lookup_n-D  NumberOfTableDimensions=1  BreakpointsForDimension1=IMUtime  BeginIndexSearchUsingPreviousIndexResult=on  Table=IMUframe  InterpMethod=Flat  DiagnosticForOutOfRangeInput=Error  RndMeth=Simplest  InputSameDT=on
  Mux5 : Mux  Inputs=3
  Mux7 : Mux  Inputs=2
  Pitch : Lookup_n-D  NumberOfTableDimensions=1  BreakpointsForDimension1=ATTframe  BeginIndexSearchUsingPreviousIndexResult=on  Table=Pitch  InterpMethod=Flat  OutDataTypeStr=single  RndMeth=Simplest  InputSameDT=on
  Roll : Lookup_n-D  NumberOfTableDimensions=1  BreakpointsForDimension1=ATTframe  BeginIndexSearchUsingPreviousIndexResult=on  Table=Roll  InterpMethod=Flat  OutDataTypeStr=single  RndMeth=Simplest  InputSameDT=on
  Velocity Down : Lookup_n-D  NumberOfTableDimensions=1  BreakpointsForDimension1=GPSframe  BeginIndexSearchUsingPreviousIndexResult=on  Table=VelD  InterpMethod=Flat  OutDataTypeStr=single  RndMeth=Simplest  InputSameDT=on
  Yaw : Lookup_n-D  NumberOfTableDimensions=1  BreakpointsForDimension1=ATTframe  BeginIndexSearchUsingPreviousIndexResult=on  Table=Yaw  InterpMethod=Flat  OutDataTypeStr=single  RndMeth=Simplest  InputSameDT=on
  wrapAng to +-pi : Subsystem
  EulAHRS : Outport  OutDataTypeStr=single
  HgtMea : Outport  Port=2  OutDataTypeStr=single
  LatLongDeg : Outport  Port=3  OutDataTypeStr=single
  GndSpd : Outport  Port=4  OutDataTypeStr=single
  CourseDeg : Outport  Port=5  OutDataTypeStr=single
  VelD : Outport  Port=6  OutDataTypeStr=single
  wires:
  Lookup Frame Counter/1 -> Ground Speed/1, Ground Course/1, Velocity Down/1, Hgt/1, LngDeg/1, LatDeg/1, Roll/1, Pitch/1, Yaw/1
  Velocity Down/1 -> VelD/1
  Roll/1 -> Mux5/1
  Pitch/1 -> Mux5/2
  Yaw/1 -> wrapAng to +-pi/1(In1)
  Mux5/1 -> EulAHRS/1
  wrapAng to +-pi/1(Out1) -> Mux5/3
  time/1 -> Lookup Frame Counter/1
  LatDeg/1 -> Mux7/1
  LngDeg/1 -> Mux7/2
  Mux7/1 -> LatLongDeg/1
  Ground Speed/1 -> GndSpd/1
  Ground Course/1 -> CourseDeg/1
  Hgt/1 -> HgtMea/1

== system NavFilterTestHarness24/LogData/Quat2Eul ==
  Quat : Inport  PortDimensions=4
  Mux : Mux  Inputs=3
  Pitch : Fcn  Expr=-asin(2*(u[2]*u[4]-u[1]*u[3]))
  Roll : Fcn  Expr=atan2(2*(u[3]*u[4]+u[1]*u[2] ) , u[1]^2-u[2]^2-u[3]^2+u[4]^2)
  Yaw : Fcn  Expr=atan2(2*(u[2]*u[3]+u[1]*u[4] ) , u[1]^2+u[2]^2-u[3]^2-u[4]^2)
  Eul : Outport
  wires:
  Mux/1 -> Eul/1
  Roll/1 -> Mux/1
  Pitch/1 -> Mux/2
  Quat/1 -> Roll/1, Pitch/1, Yaw/1
  Yaw/1 -> Mux/3

== system NavFilterTestHarness24/WatchDog/Get AHRS Data ==
  time : Inport
  Lookup Frame Counter : Lookup_n-D  NumberOfTableDimensions=1  BreakpointsForDimension1=IMUtime  BeginIndexSearchUsingPreviousIndexResult=on  Table=IMUframe  InterpMethod=Flat  DiagnosticForOutOfRangeInput=Error  RndMeth=Simplest  InputSameDT=on
  Mux5 : Mux  Inputs=3
  Pitch : Lookup_n-D  NumberOfTableDimensions=1  BreakpointsForDimension1=ATTframe  BeginIndexSearchUsingPreviousIndexResult=on  Table=Pitch  InterpMethod=Flat  OutDataTypeStr=single  RndMeth=Simplest  InputSameDT=on
  Roll : Lookup_n-D  NumberOfTableDimensions=1  BreakpointsForDimension1=ATTframe  BeginIndexSearchUsingPreviousIndexResult=on  Table=Roll  InterpMethod=Flat  OutDataTypeStr=single  RndMeth=Simplest  InputSameDT=on
  Yaw : Lookup_n-D  NumberOfTableDimensions=1  BreakpointsForDimension1=ATTframe  BeginIndexSearchUsingPreviousIndexResult=on  Table=Yaw  InterpMethod=Flat  OutDataTypeStr=single  RndMeth=Simplest  InputSameDT=on
  wrapAng to +-pi : Subsystem
  Out1 : Outport
  wires:
  Lookup Frame Counter/1 -> Roll/1, Pitch/1, Yaw/1
  Roll/1 -> Mux5/1
  Pitch/1 -> Mux5/2
  Yaw/1 -> wrapAng to +-pi/1(In1)
  wrapAng to +-pi/1(Out1) -> Mux5/3
  time/1 -> Lookup Frame Counter/1
  Mux5/1 -> Out1/1

== system NavFilterTestHarness24/WatchDog/Quat2Eul ==
  q : Inport  PortDimensions=4
  Mux : Mux  Inputs=3
  phi : Fcn  Expr=atan2(2*(u[3]*u[4]+u[1]*u[2] ) , u[1]^2-u[2]^2-u[3]^2+u[4]^2)
  psi : Fcn  Expr=atan2(2*(u[2]*u[3]+u[1]*u[4] ) , u[1]^2+u[2]^2-u[3]^2-u[4]^2)
  theta : Fcn  Expr=-asin(2*(u[2]*u[4]-u[1]*u[3]))
  Eul : Outport
  wires:
  Mux/1 -> Eul/1
  phi/1 -> Mux/1
  theta/1 -> Mux/2
  q/1 -> phi/1, theta/1, psi/1
  psi/1 -> Mux/3

== system NavFilterTestHarness24/InertialNavFilter/CalculateInitialStates/Eul2Quat ==
  Eul : Inport
  Gain : Gain  Gain=0.5  SaturateOnIntegerOverflow=on  OutDataTypeStr=Inherit: Same as input  ParamDataTypeStr=Inherit: Same as input
  Mux : Mux
  Mux1 : Mux  Inputs=[3 3]
  cos(0.5*E) : Trigonometry  Operator=cos
  q0 : Fcn  Expr=u[1] * u[2] * u[3] + u[4] * u[5] * u[6]
  q1 : Fcn  Expr=u[4] * u[2] * u[3] - u[1] * u[5] * u[6]
  q2 : Fcn  Expr=u[1] * u[5] * u[3] + u[4] * u[2] * u[6]
  q3 : Fcn  Expr=u[1] * u[2] * u[6] - u[4] * u[5] * u[3]
  sin(0.5*E)1 : Trigonometry
  Quat : Outport
  wires:
  Eul/1 -> Gain/1
  Gain/1 -> cos(0.5*E)/1, sin(0.5*E)1/1
  cos(0.5*E)/1 -> Mux1/1
  sin(0.5*E)1/1 -> Mux1/2
  q0/1 -> Mux/1
  Mux/1 -> Quat/1
  q1/1 -> Mux/2
  q2/1 -> Mux/3
  q3/1 -> Mux/4
  Mux1/1 -> q0/1, q1/1, q3/1, q2/1

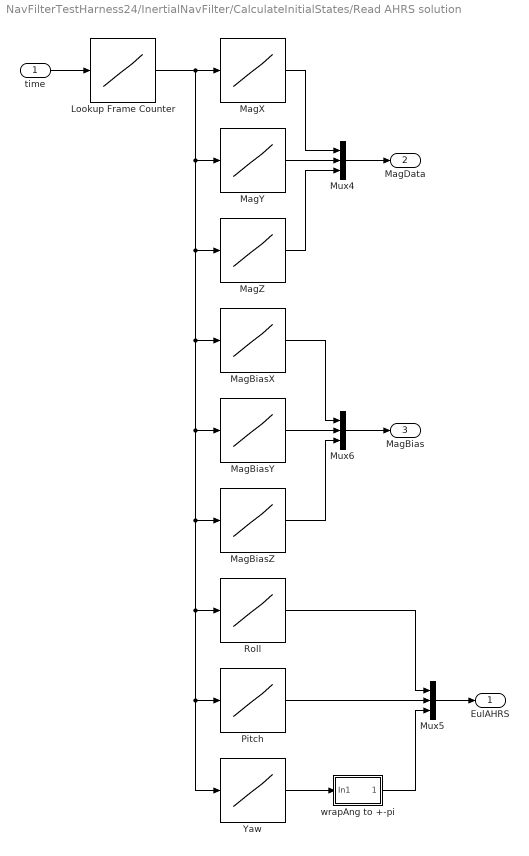
== system NavFilterTestHarness24/InertialNavFilter/CalculateInitialStates/Read AHRS solution ==
  time : Inport
  Lookup Frame Counter : Lookup_n-D  NumberOfTableDimensions=1  BreakpointsForDimension1=IMUtime  BeginIndexSearchUsingPreviousIndexResult=on  Table=IMUframe  InterpMethod=Flat  DiagnosticForOutOfRangeInput=Error  RndMeth=Simplest  InputSameDT=on
  MagBiasX : Lookup_n-D  NumberOfTableDimensions=1  BreakpointsForDimension1=MAGframe  BeginIndexSearchUsingPreviousIndexResult=on  Table=MagBiasX  InterpMethod=Flat  OutDataTypeStr=single  RndMeth=Simplest  InputSameDT=on
  MagBiasY : Lookup_n-D  NumberOfTableDimensions=1  BreakpointsForDimension1=MAGframe  BeginIndexSearchUsingPreviousIndexResult=on  Table=MagBiasY  InterpMethod=Flat  OutDataTypeStr=single  RndMeth=Simplest  InputSameDT=on
  MagBiasZ : Lookup_n-D  NumberOfTableDimensions=1  BreakpointsForDimension1=MAGframe  BeginIndexSearchUsingPreviousIndexResult=on  Table=MagBiasZ  InterpMethod=Flat  OutDataTypeStr=single  RndMeth=Simplest  InputSameDT=on
  MagX : Lookup_n-D  NumberOfTableDimensions=1  BreakpointsForDimension1=MAGframe  BeginIndexSearchUsingPreviousIndexResult=on  Table=MagX  InterpMethod=Flat  OutDataTypeStr=single  RndMeth=Simplest  InputSameDT=on
  MagY : Lookup_n-D  NumberOfTableDimensions=1  BreakpointsForDimension1=MAGframe  BeginIndexSearchUsingPreviousIndexResult=on  Table=MagY  InterpMethod=Flat  OutDataTypeStr=single  RndMeth=Simplest  InputSameDT=on
  MagZ : Lookup_n-D  NumberOfTableDimensions=1  BreakpointsForDimension1=MAGframe  BeginIndexSearchUsingPreviousIndexResult=on  Table=MagZ  InterpMethod=Flat  OutDataTypeStr=single  RndMeth=Simplest  InputSameDT=on
  Mux4 : Mux  Inputs=3
  Mux5 : Mux  Inputs=3
  Mux6 : Mux  Inputs=3
  Pitch : Lookup_n-D  NumberOfTableDimensions=1  BreakpointsForDimension1=ATTframe  BeginIndexSearchUsingPreviousIndexResult=on  Table=Pitch  InterpMethod=Flat  OutDataTypeStr=single  RndMeth=Simplest  InputSameDT=on
  Roll : Lookup_n-D  NumberOfTableDimensions=1  BreakpointsForDimension1=ATTframe  BeginIndexSearchUsingPreviousIndexResult=on  Table=Roll  InterpMethod=Flat  OutDataTypeStr=single  RndMeth=Simplest  InputSameDT=on
  Yaw : Lookup_n-D  NumberOfTableDimensions=1  BreakpointsForDimension1=ATTframe  BeginIndexSearchUsingPreviousIndexResult=on  Table=Yaw  InterpMethod=Flat  OutDataTypeStr=single  RndMeth=Simplest  InputSameDT=on
  wrapAng to +-pi : Subsystem
  EulAHRS : Outport  OutDataTypeStr=single
  MagData : Outport  Port=2  OutDataTypeStr=single
  MagBias : Outport  Port=3  OutDataTypeStr=single
  wires:
  Lookup Frame Counter/1 -> MagX/1, MagY/1, MagZ/1, MagBiasX/1, MagBiasY/1, MagBiasZ/1, Roll/1, Yaw/1, Pitch/1
  Mux4/1 -> MagData/1
  MagY/1 -> Mux4/2
  MagX/1 -> Mux4/1
  MagZ/1 -> Mux4/3
  time/1 -> Lookup Frame Counter/1
  Mux6/1 -> MagBias/1
  MagBiasY/1 -> Mux6/2
  MagBiasX/1 -> Mux6/1
  MagBiasZ/1 -> Mux6/3
  Roll/1 -> Mux5/1
  Pitch/1 -> Mux5/2
  Yaw/1 -> wrapAng to +-pi/1(In1)
  Mux5/1 -> EulAHRS/1
  wrapAng to +-pi/1(Out1) -> Mux5/3

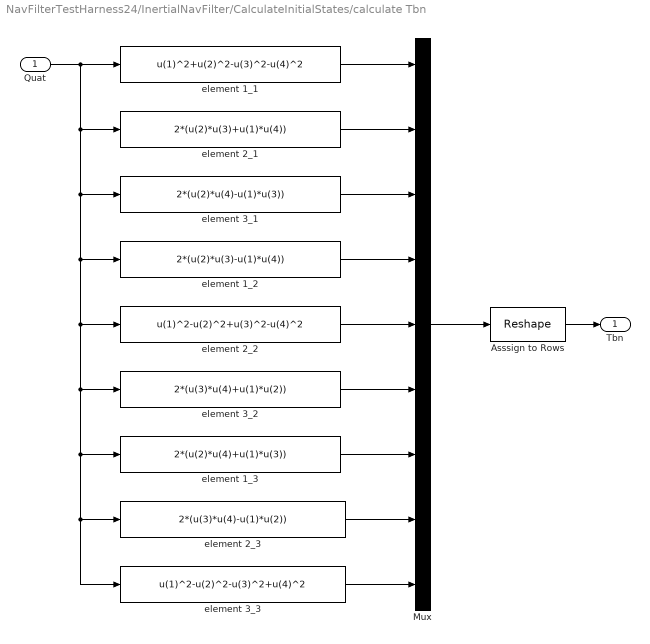
== system NavFilterTestHarness24/InertialNavFilter/CalculateInitialStates/calculate Tbn ==
  Quat : Inport  PortDimensions=4
  Asssign to Rows : Reshape  OutputDimensionality=Customize  OutputDimensions=[3,3]
  Mux : Mux  Inputs=9
  element 1_1 : Fcn  Expr=u(1)^2+u(2)^2-u(3)^2-u(4)^2
  element 1_2 : Fcn  Expr=2*(u(2)*u(3)-u(1)*u(4))
  element 1_3 : Fcn  Expr=2*(u(2)*u(4)+u(1)*u(3))
  element 2_1 : Fcn  Expr=2*(u(2)*u(3)+u(1)*u(4))
  element 2_2 : Fcn  Expr=u(1)^2-u(2)^2+u(3)^2-u(4)^2
  element 2_3 : Fcn  Expr=2*(u(3)*u(4)-u(1)*u(2))
  element 3_1 : Fcn  Expr=2*(u(2)*u(4)-u(1)*u(3))
  element 3_2 : Fcn  Expr=2*(u(3)*u(4)+u(1)*u(2))
  element 3_3 : Fcn  Expr=u(1)^2-u(2)^2-u(3)^2+u(4)^2
  Tbn : Outport
  wires:
  Mux/1 -> Asssign to Rows/1
  element 1_1/1 -> Mux/1
  element 2_1/1 -> Mux/2
  element 3_1/1 -> Mux/3
  element 1_2/1 -> Mux/4
  element 2_2/1 -> Mux/5
  element 3_2/1 -> Mux/6
  element 1_3/1 -> Mux/7
  element 2_3/1 -> Mux/8
  element 3_3/1 -> Mux/9
  Asssign to Rows/1 -> Tbn/1
  Quat/1 -> element 1_1/1, element 3_3/1, element 2_3/1, element 1_3/1, element 3_2/1, element 2_2/1, element 1_2/1, element 3_1/1, element 2_1/1

== system NavFilterTestHarness24/InertialNavFilter/Log Internal Data/Log Airspeed Innovations ==
  innovation : Inport
  varInnov : Inport  Port=2
  time : Inport  Port=3
  Trigger : TriggerPort  VariantControl=Variant  PortDimensions=1
  Gain : Gain  Gain=-1
  Mux : Mux  Inputs=3
  Sqrt : Sqrt  SaturateOnIntegerOverflow=on
  To Workspace : ToWorkspace  VariableName=innovVtas  SampleTime=-1
  To Workspace6 : ToWorkspace  VariableName=time3  SampleTime=-1
  wires:
  Mux/1 -> To Workspace/1  "Vtas innovation"
  innovation/1 -> Mux/1  "Vtas innovation"
  varInnov/1 -> Sqrt/1
  Sqrt/1 -> Mux/2, Gain/1
  Gain/1 -> Mux/3
  time/1 -> To Workspace6/1

== system NavFilterTestHarness24/InertialNavFilter/Log Internal Data/Log MagX Innovations ==
  innovation : Inport
  varInnov : Inport  Port=2
  time : Inport  Port=3
  Trigger : TriggerPort  VariantControl=Variant  PortDimensions=1
  Gain : Gain  Gain=-1
  Mux : Mux  Inputs=3
  Selector : Selector  InputPortWidth=3  IndexOptions=Index vector (dialog)  Indices=1  OutputSizes=1
  Selector1 : Selector  InputPortWidth=3  IndexOptions=Index vector (dialog)  Indices=1  OutputSizes=1
  Selector2 : Selector  InputPortWidth=3  IndexOptions=Index vector (dialog)  Indices=1  OutputSizes=1
  Sqrt : Sqrt  SaturateOnIntegerOverflow=on
  To Workspace : ToWorkspace  VariableName=innovMagX  SampleTime=-1
  To Workspace6 : ToWorkspace  VariableName=time2  SampleTime=-1
  wires:
  Mux/1 -> To Workspace/1  "MagX innovation"
  Gain/1 -> Selector1/1
  Sqrt/1 -> Gain/1, Selector/1
  varInnov/1 -> Sqrt/1
  innovation/1 -> Selector2/1
  time/1 -> To Workspace6/1
  Selector/1 -> Mux/2
  Selector1/1 -> Mux/3
  Selector2/1 -> Mux/1

== system NavFilterTestHarness24/InertialNavFilter/Log Internal Data/Log MagY Innovations ==
  innovation : Inport
  varInnov : Inport  Port=2
  Trigger : TriggerPort  VariantControl=Variant  PortDimensions=1
  Gain : Gain  Gain=-1
  Mux1 : Mux  Inputs=3
  Selector1 : Selector  InputPortWidth=3  IndexOptions=Index vector (dialog)  Indices=2  OutputSizes=1
  Selector2 : Selector  InputPortWidth=3  IndexOptions=Index vector (dialog)  Indices=2  OutputSizes=1
  Selector3 : Selector  InputPortWidth=3  IndexOptions=Index vector (dialog)  Indices=2  OutputSizes=1
  Sqrt : Sqrt  SaturateOnIntegerOverflow=on
  To Workspace1 : ToWorkspace  VariableName=innovMagY  SampleTime=-1
  wires:
  Mux1/1 -> To Workspace1/1  "MagY innovation"
  Gain/1 -> Selector3/1
  Sqrt/1 -> Gain/1, Selector2/1
  varInnov/1 -> Sqrt/1
  innovation/1 -> Selector1/1
  Selector1/1 -> Mux1/1
  Selector2/1 -> Mux1/2
  Selector3/1 -> Mux1/3

== system NavFilterTestHarness24/InertialNavFilter/Log Internal Data/Log MagZ Innovations ==
  innovation : Inport
  varInnov : Inport  Port=2
  Trigger : TriggerPort  VariantControl=Variant  PortDimensions=1
  Gain : Gain  Gain=-1
  Mux2 : Mux  Inputs=3
  Selector1 : Selector  InputPortWidth=3  IndexOptions=Index vector (dialog)  Indices=3  OutputSizes=1
  Selector2 : Selector  InputPortWidth=3  IndexOptions=Index vector (dialog)  Indices=3  OutputSizes=1
  Selector3 : Selector  InputPortWidth=3  IndexOptions=Index vector (dialog)  Indices=3  OutputSizes=1
  Sqrt : Sqrt  SaturateOnIntegerOverflow=on
  To Workspace2 : ToWorkspace  VariableName=innovMagZ  SampleTime=-1
  wires:
  Mux2/1 -> To Workspace2/1  "MagZ innovation"
  Gain/1 -> Selector3/1
  Sqrt/1 -> Gain/1, Selector2/1
  varInnov/1 -> Sqrt/1
  innovation/1 -> Selector1/1
  Selector1/1 -> Mux2/1
  Selector2/1 -> Mux2/2
  Selector3/1 -> Mux2/3

== system NavFilterTestHarness24/InertialNavFilter/Log Internal Data/Log PosD Innovations ==
  innovation : Inport
  varInnov : Inport  Port=2
  time : Inport  Port=3
  Trigger : TriggerPort  VariantControl=Variant  PortDimensions=1
  Gain : Gain  Gain=-1
  Mux5 : Mux  Inputs=3
  Selector : Selector  InputPortWidth=6  IndexOptions=Index vector (dialog)  Indices=6  OutputSizes=1
  Selector1 : Selector  InputPortWidth=6  IndexOptions=Index vector (dialog)  Indices=6  OutputSizes=1
  Selector2 : Selector  InputPortWidth=6  IndexOptions=Index vector (dialog)  Indices=6  OutputSizes=1
  Sqrt : Sqrt  SaturateOnIntegerOverflow=on
  To Workspace5 : ToWorkspace  VariableName=innovPosD  SampleTime=-1
  To Workspace6 : ToWorkspace  VariableName=time4  SampleTime=-1
  wires:
  time/1 -> To Workspace6/1
  Mux5/1 -> To Workspace5/1  "PosD innovation"
  Selector1/1 -> Mux5/2
  Selector/1 -> Mux5/1  "PosD innovation"
  Gain/1 -> Selector2/1
  Sqrt/1 -> Gain/1, Selector1/1
  varInnov/1 -> Sqrt/1
  innovation/1 -> Selector/1
  Selector2/1 -> Mux5/3

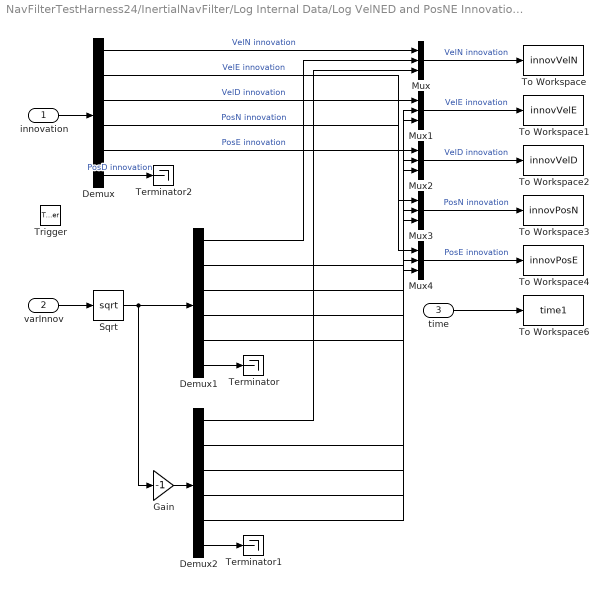
== system NavFilterTestHarness24/InertialNavFilter/Log Internal Data/Log VelNED and PosNE Innovations ==
  innovation : Inport
  varInnov : Inport  Port=2
  time : Inport  Port=3
  Trigger : TriggerPort  VariantControl=Variant  PortDimensions=1
  Demux : Demux  Outputs=6
  Demux1 : Demux  Outputs=6
  Demux2 : Demux  Outputs=6
  Gain : Gain  Gain=-1
  Mux{,1..4} (5 alike) : Mux  Inputs=3
  Sqrt : Sqrt  SaturateOnIntegerOverflow=on
  Terminator : Terminator
  Terminator1 : Terminator
  Terminator2 : Terminator
  To Workspace : ToWorkspace  VariableName=innovVelN  SampleTime=-1
  To Workspace1 : ToWorkspace  VariableName=innovVelE  SampleTime=-1
  To Workspace2 : ToWorkspace  VariableName=innovVelD  SampleTime=-1
  To Workspace3 : ToWorkspace  VariableName=innovPosN  SampleTime=-1
  To Workspace4 : ToWorkspace  VariableName=innovPosE  SampleTime=-1
  To Workspace6 : ToWorkspace  VariableName=time1  SampleTime=-1
  wires:
  innovation/1 -> Demux/1
  varInnov/1 -> Sqrt/1
  Sqrt/1 -> Demux1/1, Gain/1
  Gain/1 -> Demux2/1
  Demux/1 -> Mux/1  "VelN innovation"
  Demux1/1 -> Mux/2
  Demux2/1 -> Mux/3
  Demux/2 -> Mux1/1  "VelE innovation"
  Demux1/2 -> Mux1/2
  Demux2/2 -> Mux1/3
  Demux/3 -> Mux2/1  "VelD innovation"
  Demux1/3 -> Mux2/2
  Demux2/3 -> Mux2/3
  Demux/4 -> Mux3/1  "PosN innovation"
  Demux1/4 -> Mux3/2
  Demux2/4 -> Mux3/3
  Demux/5 -> Mux4/1  "PosE innovation"
  Demux1/5 -> Mux4/2
  Demux2/5 -> Mux4/3
  Mux/1 -> To Workspace/1  "VelN innovation"
  Mux1/1 -> To Workspace1/1  "VelE innovation"
  Mux2/1 -> To Workspace2/1  "VelD innovation"
  Mux3/1 -> To Workspace3/1  "PosN innovation"
  Mux4/1 -> To Workspace4/1  "PosE innovation"
  time/1 -> To Workspace6/1
  Demux1/6 -> Terminator/1
  Demux2/6 -> Terminator1/1
  Demux/6 -> Terminator2/1  "PosD innovation"
